simulink model "PowerControlUnit"  (R2024a)
settings: Solver=VariableStepAuto  StartTime=0.0  StopTime=10.0  RelTol=1e-3
libraries: aerolibactuator x4
settings Model: Creator=chico  LastModifiedBy=chico

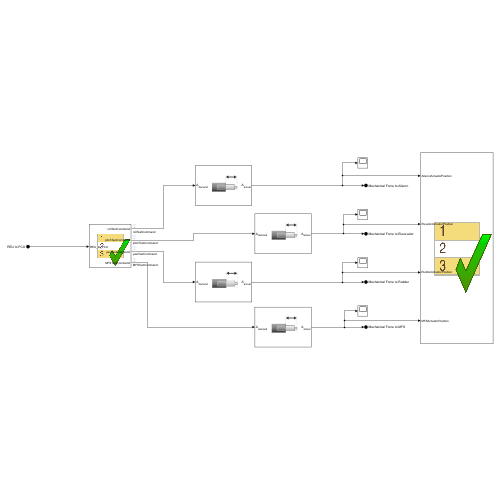
[thumbnail: Simulink's stored preview of the top-level diagram]
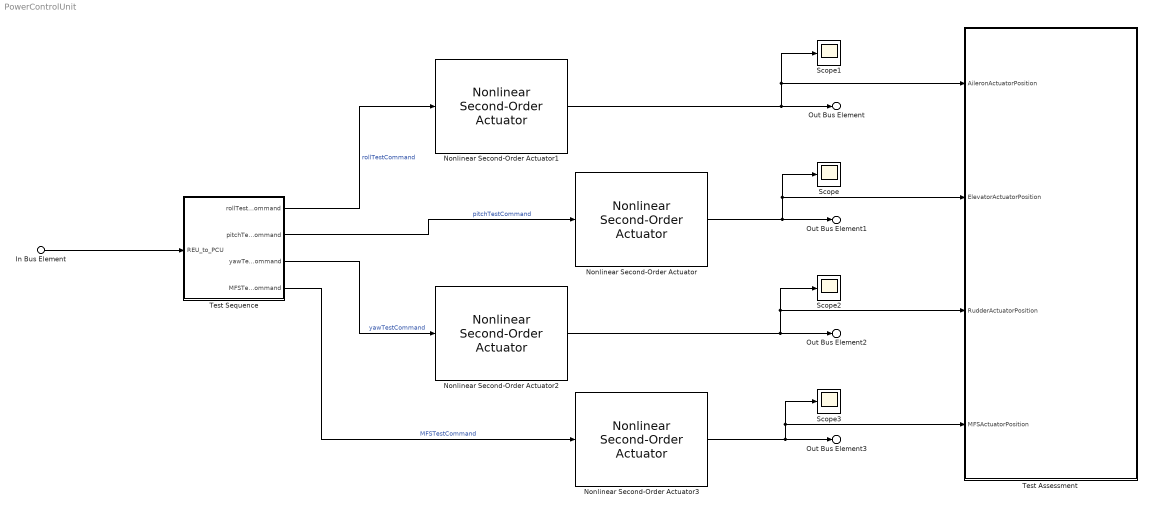
== system PowerControlUnit ==
  In Bus Element : Inport  PortName=REU to PCU
  Nonlinear Second-Order Actuator : aerolibactuator/Nonlinear Second-Order Actuator  wn_fin=1  z_fin=0.3  fin_max=10  fin_min=-10  fin_maxrate=500*pi/180  fin_act_0=0  fin_act_vel=0
  Nonlinear Second-Order Actuator1 : aerolibactuator/Nonlinear Second-Order Actuator  wn_fin=1  z_fin=0.3  fin_max=10  fin_min=-10  fin_maxrate=500*pi/180  fin_act_0=0  fin_act_vel=0
  Nonlinear Second-Order Actuator2 : aerolibactuator/Nonlinear Second-Order Actuator  wn_fin=1  z_fin=0.3  fin_max=15  fin_min=-15  fin_maxrate=500*pi/180  fin_act_0=0  fin_act_vel=0
  Nonlinear Second-Order Actuator3 : aerolibactuator/Nonlinear Second-Order Actuator  wn_fin=1  z_fin=0.3  fin_max=10  fin_min=-10  fin_maxrate=500*pi/180  fin_act_0=0  fin_act_vel=0
  Scope{,1..3} (4 alike) : Scope
  Test Assessment : Test Sequence  TreatAsAtomicUnit=on
  Test Sequence : Test Sequence  TreatAsAtomicUnit=on
  Out Bus Element : Outport  PortName=Mechanical Force to Aileron
  Out Bus Element1 : Outport  Port=2  PortName=Mechanical Force to Elevevator
  Out Bus Element2 : Outport  Port=3  PortName=Mechanical Force to Rudder
  Out Bus Element3 : Outport  Port=4  PortName=Mechanical Force to MFS
  wires:
  Nonlinear Second-Order Actuator2/1 -> Out Bus Element2/1, Scope2/1, Test Assessment/3(RudderActuatorPosition)
  Nonlinear Second-Order Actuator1/1 -> Out Bus Element/1, Scope1/1, Test Assessment/1(AileronActuatorPosition)
  Nonlinear Second-Order Actuator/1 -> Out Bus Element1/1, Scope/1, Test Assessment/2(ElevatorActuatorPosition)
  Nonlinear Second-Order Actuator3/1 -> Out Bus Element3/1, Scope3/1, Test Assessment/4(MFSActuatorPosition)
  In Bus Element/1 -> Test Sequence/1(REU_to_PCU)
  Test Sequence/1(rollTestCommand) -> Nonlinear Second-Order Actuator1/1  "rollTestCommand"
  Test Sequence/2(pitchTestCommand) -> Nonlinear Second-Order Actuator/1  "pitchTestCommand"
  Test Sequence/3(yawTestCommand) -> Nonlinear Second-Order Actuator2/1  "yawTestCommand"
  Test Sequence/4(MFSTestCommand) -> Nonlinear Second-Order Actuator3/1  "MFSTestCommand"

== stateflow chart PowerControlUnit/Test Assessment ==
  state step_1
    assert(0==0)
    state step_1_1
      verify(AileronActuatorPosition <= 10 && AileronActuatorPosition >= -10)
      verify(ElevatorActuatorPosition <= 10 && ElevatorActuatorPosition >= -10)
      verify(RudderActuatorPosition <= 10 && RudderActuatorPosition >= -10)
      verify(MFSActuatorPosition <= 10 && MFSActuatorPosition >= -10)
    (default) -> step_1_1
  (default) -> step_1
  data: AileronActuatorPosition input; ElevatorActuatorPosition input; RudderActuatorPosition input; MFSActuatorPosition input

== stateflow chart PowerControlUnit/Test Sequence ==
  state Start
    pitchTestCommand = 0;
    rollTestCommand = 0;
    yawTestCommand = 0;
    MFSTestCommand = 0;
  state HighCommand_1
    pitchTestCommand = 11;
    rollTestCommand = 11;
    yawTestCommand = 11;
  state MiddleCommand_1
    pitchTestCommand = -5;
    rollTestCommand = -5;
    yawTestCommand = -5;
  state HighCommand_2
    pitchTestCommand = 9;
    rollTestCommand = 9;
    yawTestCommand = 9;
  state MiddleCommand_2
    pitchTestCommand = 0;
    rollTestCommand = 0;
    yawTestCommand = 0;
  state LowCommand_1
    pitchTestCommand = -11
    rollTestCommand = -11;
    yawTestCommand = -11;
  state MiddleCommand_3
    pitchTestCommand = 5;
    rollTestCommand = 5;
    yawTestCommand = 5;
  state LowCommand_2
    pitchTestCommand = -9.5
    rollTestCommand = -9.5;
    yawTestCommand = -9.5;
  state Stop
    pitchTestCommand = 0;
    rollTestCommand = 0;
    yawTestCommand = 0;
  (default) -> Start
  Start -> HighCommand_1 : [
      | after(10, sec)
      | ]
  HighCommand_1 -> MiddleCommand_1 : [
      | after(10, sec)
      | ]
  MiddleCommand_1 -> HighCommand_2 : [
      | after(10, sec)
      | ]
  HighCommand_2 -> MiddleCommand_2 : [
      | after(10, sec)
      | ]
  MiddleCommand_2 -> LowCommand_1 : [
      | after(10, sec)
      | ]
  LowCommand_1 -> MiddleCommand_3 : [
      | after(10, sec)
      | ]
  MiddleCommand_3 -> LowCommand_2 : [
      | after(10, sec)
      | ]
  LowCommand_2 -> Stop : [
      | after(10, sec)
      | ]
  data: rollTestCommand output; pitchTestCommand output; yawTestCommand output; MFSTestCommand output; REU_to_PCU input
